simulink model "num3"  (R2019a)
settings: Solver=VariableStepAuto  StartTime=0.0  StopTime=10.0  RelTol=1e-3
libraries: simulink x1
settings Model: Creator=julia  LastModifiedBy=julia

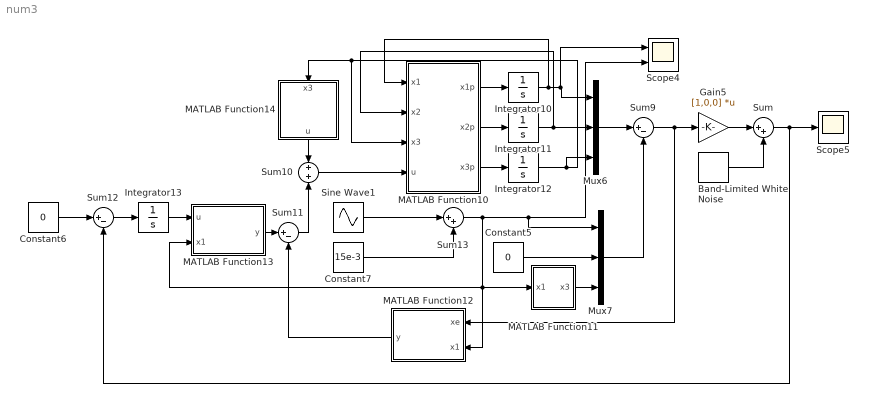
== system num3 ==
  Band-Limited White Noise : simulink/Sources/Band-Limited White Noise  Cov=[0.0000001]  Ts=0.1  seed=[23341]
  Constant5 : Constant  Value=0
  Constant6 : Constant  Value=0
  Constant7 : Constant  Value=15e-3
  Gain5 : Gain  Gain=[1,0,0]  Multiplication=Matrix(K*u)
  Integrator10 : Integrator  InitialCondition=5e-3
  Integrator11 : Integrator
  Integrator12 : Integrator
  Integrator13 : Integrator
  MATLAB Function10 : MATLAB Function  TreatAsAtomicUnit=on
  MATLAB Function11 : MATLAB Function  TreatAsAtomicUnit=on
  MATLAB Function12 : MATLAB Function  TreatAsAtomicUnit=on
  MATLAB Function13 : MATLAB Function  TreatAsAtomicUnit=on
  MATLAB Function14 : MATLAB Function  TreatAsAtomicUnit=on
  Mux6 : Mux  Inputs=3
  Mux7 : Mux  Inputs=3
  Scope4 : Scope  NumInputPorts=2
  Scope5 : Scope
  Sine Wave1 : Sin  Amplitude=10e-3  Frequency=2  Phase=3+pi/2  SampleTime=0
  Sum : Sum  Inputs=|++
  Sum10 : Sum  Inputs=+|+
  Sum11 : Sum  Inputs=|+-
  Sum12 : Sum  Inputs=|+-
  Sum13 : Sum  Inputs=|++
  Sum9 : Sum  Inputs=|+-
  wires:
  Sine Wave1/1 -> Sum13/1
  Constant7/1 -> Sum13/2
  MATLAB Function10/1(x1p) -> Integrator10/1
  MATLAB Function10/2(x2p) -> Integrator11/1
  MATLAB Function10/3(x3p) -> Integrator12/1
  Integrator10/1 -> MATLAB Function10/1(x1), Scope4/1, Mux6/1
  Integrator11/1 -> MATLAB Function10/2(x2), Mux6/2
  Integrator12/1 -> MATLAB Function14/1(x3), MATLAB Function10/3(x3), Mux6/3
  Mux6/1 -> Sum9/1
  Constant5/1 -> Mux7/2
  Sum13/1 -> MATLAB Function11/1(x1), MATLAB Function13/2(x1), MATLAB Function12/2(x1), Scope4/2, Mux7/1
  MATLAB Function11/1(x3) -> Mux7/3
  Mux7/1 -> Sum9/2
  Sum10/1 -> MATLAB Function10/4(u)
  MATLAB Function14/1(u) -> Sum10/1
  MATLAB Function13/1(y) -> Sum11/1
  Sum12/1 -> Integrator13/1
  Sum11/1 -> Sum10/2
  Sum9/1 -> MATLAB Function12/1(xe), Gain5/1
  Constant6/1 -> Sum12/1
  Integrator13/1 -> MATLAB Function13/1(u)
  MATLAB Function12/1(y) -> Sum11/2
  Gain5/1 -> Sum/1
  Sum/1 -> Sum12/2, Scope5/1
  Band-Limited White Noise/1 -> Sum/2

== matlab function num3/MATLAB Function10 ==
  data: x1 input size=1; x1p output size=1; x2 input size=1; x3 input size=1; x2p output size=1; x3p output size=1; u input size=1
function [x1p,x2p,x3p] = planta(x1,x2,x3,u)
c=0.1;
m=0.01;
L=100e-3;
r=10;
g=9.81;

x1p=x2;
x2p=g-(c/m)*((x3^2)/x1);
x3p=-(r/L)*x3+(1/L)*u;

== matlab function num3/MATLAB Function11 ==
  data: x1 input size=1; x3 output size=1
function x3  = fcn(x1)
c=1
m=0.1
L=0.01
r=1
g=9.81

x3=sqrt((m*g*x1)/c);

== matlab function num3/MATLAB Function12 ==
  data: xe input size=3; x1 input size=1; y output size=1
function y  = Kservo(xe,x1)

k1=-((2.9104e-15)*((6.1932e16)*x1+(1.6179e15)))/(sqrt(0.981*x1));
k2=-((9.0949e-17)*((1.6551e17)*x1+(5.3931e14)))/(sqrt(0.981*x1));
k3=-0.4;
k=[k1,k2,k3];
y = k*xe;

== matlab function num3/MATLAB Function13 ==
  data: u input size=1; x1 input size=1; y output size=1
function y = ki(u,x1)

k=-((1.0449e3)*x1)/(sqrt(0.981*x1));
y = k*u;

== matlab function num3/MATLAB Function14 ==
  data: x3 input size=1; u output size=1
function u  = u(x3)
c=1
m=0.1
L=0.01
r=1
g=9.81

u=r*x3;
